simulink model "dirdyna_coman_robotran"  (Simulink 8.3)
settings: Solver=ode4  StartTime=0  StopTime=60  FixedStep=0.0005  MaxStep=1e-2  RelTol=1e-3  AbsTol=1e-6
undefined symbols (not defined in the file or in its folder): Function_dirdynared, MBStoAnimFile_StopFcnCallback, Modules, Robotran, S
settings Model: Creator=nvandernoot  LastModifiedBy=nico
settings SolverCC: InitialStep=1e-3
settings OptimizationCC: ExpressionDepthLimit=2147483647
settings DebuggingCC: FcnCallInpInsideContextMsg=UseLocalSettings

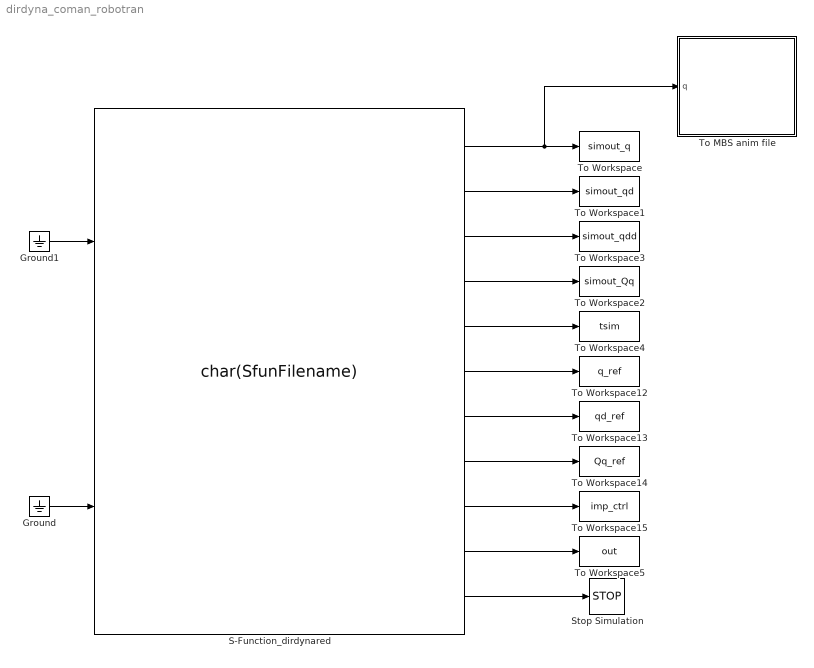
== system dirdyna_coman_robotran ==
  Ground : Ground
  Ground1 : Ground
  S-Function_dirdynared : S-Function  AncestorBlock=Robotran/Modules/S-Function_dirdynared  FunctionName=char(SfunFilename)  Parameters=getfield(get(gcbh,'UserData'),'mbs_data') q_ini  EnableBusSupport=off  mask(S-function: Robotran Direct Dynamics (dirdynared)){SfunFilename=mbs_sf_dirdynared_coman_robotran, q_ini=off, creation_date=29-Oct-2013}
      mask prompts: SfunFilename "S-function filename"; q_ini "Get initial qu from block inputs"; creation_date "Enter the creation date:"
      mask help: Compute the Direct Dynamics equations using symbolic MBS formalism
      settings: OpenFcn=MBSdirdynaredSfunction
      settings: CopyFcn=|
      | MBSdirdynaredSfunction;
      | set_param(gcs,'MaxStep','1e-2');
      | set_param(gcs,'InitialStep','1e-3');
      | set_param(gcs,'RelTol','1e-3');
      | set_param(gcs,'AbsTol','1e-6');
      | set_param(gcb,'OpenFcn','MBSdirdynaredSfunction');
      | set_param(gcb,'creation_date',date);
      mask Display:
      | disp('Robotran\nDirect\nDynamics\n(dirdynared)\n-\n coman_robotran\n-\n29-Oct-2013');
      | port_label('input',1,'Joint forces');
      | port_label('input',2,'Driven joints');
      | port_label('output',1,'q');
      | port_label('output',2,'qd');
      | port_label('output',3,'qdd');
  Stop Simulation : Stop
  To MBS anim file : Subsystem  AncestorBlock=Robotran/Utilities/To MBS anim file  StopFcn=MBStoAnimFile_StopFcnCallback;  mask{varname=tqres, filename=simdir.anim, prjname=coman_robotran, overwrite=0, samplingRate=1000}
      mask prompts: varname "variable name"; filename "anim file name"; prjname "project name"; samplingRate "sampling rate"
      settings: CopyFcn=MBStoAnimFile_v2;  OpenFcn=MBStoAnimFile_v2;
      mask Display: image(imread('Logo_anim.jpg'))
  To Workspace : ToWorkspace  VariableName=simout_q  SaveFormat=Structure  SampleTime=-1
  To Workspace1 : ToWorkspace  VariableName=simout_qd  SaveFormat=Structure  SampleTime=-1
  To Workspace12 : ToWorkspace  VariableName=q_ref  SaveFormat=Structure  SampleTime=-1
  To Workspace13 : ToWorkspace  VariableName=qd_ref  SaveFormat=Structure  SampleTime=-1
  To Workspace14 : ToWorkspace  VariableName=Qq_ref  SaveFormat=Structure  SampleTime=-1
  To Workspace15 : ToWorkspace  VariableName=imp_ctrl  SaveFormat=Structure  SampleTime=-1
  To Workspace2 : ToWorkspace  VariableName=simout_Qq  SaveFormat=Structure  SampleTime=-1
  To Workspace3 : ToWorkspace  VariableName=simout_qdd  SaveFormat=Structure  SampleTime=-1
  To Workspace4 : ToWorkspace  VariableName=tsim  SaveFormat=Structure  SampleTime=-1
  To Workspace5 : ToWorkspace  VariableName=out  SaveFormat=Structure  SampleTime=-1
  wires:
  Ground1/1 -> S-Function_dirdynared/1
  Ground/1 -> S-Function_dirdynared/2
  S-Function_dirdynared/1 -> To MBS anim file/1(q), To Workspace/1
  S-Function_dirdynared/2 -> To Workspace1/1
  S-Function_dirdynared/3 -> To Workspace3/1
  S-Function_dirdynared/4 -> To Workspace2/1
  S-Function_dirdynared/5 -> To Workspace4/1
  S-Function_dirdynared/6 -> To Workspace12/1
  S-Function_dirdynared/7 -> To Workspace13/1
  S-Function_dirdynared/8 -> To Workspace14/1
  S-Function_dirdynared/9 -> To Workspace15/1
  S-Function_dirdynared/10 -> To Workspace5/1
  S-Function_dirdynared/11 -> Stop Simulation/1

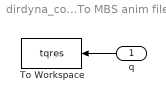
== system dirdyna_coman_robotran/To MBS anim file ==
  q : Inport
  To Workspace : ToWorkspace  VariableName=tqres  SaveFormat=Structure With Time  SampleTime=-1
  wires:
  q/1 -> To Workspace/1
